simulink model "Lab2"  (Simulink 8.8)
settings: Solver=VariableStepAuto  StartTime=0.0  StopTime=0.2  FixedStep=0.001  MaxStep=10^(-3)  RelTol=1e-3  EnableMultiTasking=on
settings Model: Creator=student  LastModifiedBy=Admin
settings OptimizationCC: ExpressionDepthLimit=2147483647  InitFltsAndDblsToZero=on
settings DebuggingCC: SaveWithParameterizedLinksMsg=none  SolverPrmCheckMsg=warning
settings GRTTargetCC: TargetFcnLib=ansi_tfl_tmw.mat  GeneratePreprocessorConditionals=Use local settings

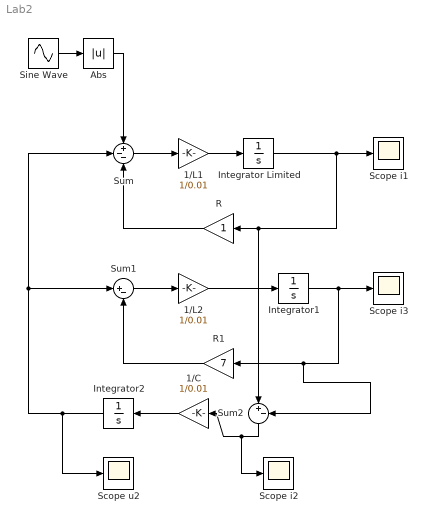
== system Lab2 ==
  1/C : Gain  Gain=1/0.01
  1/L1 : Gain  Gain=1/0.01
  1/L2 : Gain  Gain=1/0.01
  Abs : Abs
  Integrator Limited : Integrator  LimitOutput=on  LowerSaturationLimit=0
  Integrator1 : Integrator
  Integrator2 : Integrator
  R : Gain
  R1 : Gain  Gain=7
  Scope i1 : Scope
  Scope i2 : Scope
  Scope i3 : Scope
  Scope u2 : Scope
  Sine Wave : Sin  Amplitude=310  Frequency=314  SampleTime=0
  Sum : Sum  Inputs=+--
  Sum1 : Sum  Inputs=|+-
  Sum2 : Sum  Inputs=|+-
  wires:
  Sum/1 -> 1/L1/1
  Integrator Limited/1 -> Scope i1/1, Sum2/1, R/1
  R/1 -> Sum/3
  Sum1/1 -> 1/L2/1
  1/L2/1 -> Integrator1/1
  Integrator1/1 -> Scope i3/1, Sum2/2, R1/1
  R1/1 -> Sum1/2
  1/C/1 -> Integrator2/1
  Integrator2/1 -> Scope u2/1, Sum1/1, Sum/2
  Sum2/1 -> Scope i2/1, 1/C/1
  1/L1/1 -> Integrator Limited/1
  Sine Wave/1 -> Abs/1
  Abs/1 -> Sum/1
